simulink model "Adjustable_InputVoltage_Inverter"  (R2015a)
settings: Solver=ode45  StartTime=0.0  StopTime=1  RelTol=1e-3
libraries: powerlib x27, powerlib_meascontrol x7, simulink x2
settings Model: Creator=Koustubh  LastModifiedBy=Koustubh

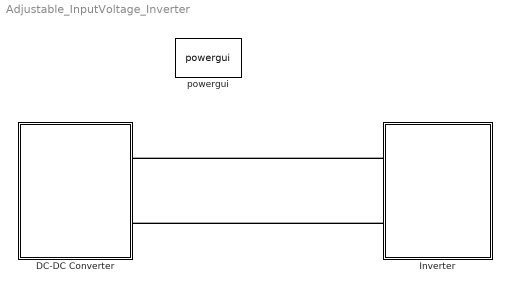
== system Adjustable_InputVoltage_Inverter ==
  DC-DC Converter : Subsystem
  Inverter : Subsystem
  powergui : powerlib/powergui  Priority=1  SimulationMode=Discrete  SolverType=Tustin/Backward Euler (TBE)  SampleTime=50e-6  frequency=60  SPID=off  DisableSnubberDevices=off  DisableRonSwitches=off  DisableVfSwitches=off  SwTol=0  DisplayEquations=off  Interpol=off  methode=off  Ts=100  FunctionMessages=off  echomessages=off  HookPort=off  EnableUseOfTLC=off  x0status=blocks  frequencyindice=0  Pbase=100e6  ErrMax=1e-4  Iterations=50  UnitsV=kV  UnitsW=MW  buscounter=0  RestoreLinks=warning  ResistiveCurrentMeasurement=off  Frange=[0:2:500]  Ylog=off  Xlog=on  ShowGrid=off  save=off  variable=ZData  structure=0  ZoomFFT=off  StartTime=0.0  cycles=1  DisplayStyle=1  fundamental=60  FreqAxis=off  MaxFrequency=1000  frequencyindicesteady=1  RmsSteady=1  display=off
  connections:
  Inverter/LConn1 -- DC-DC Converter/RConn1
  Inverter/LConn2 -- DC-DC Converter/RConn2

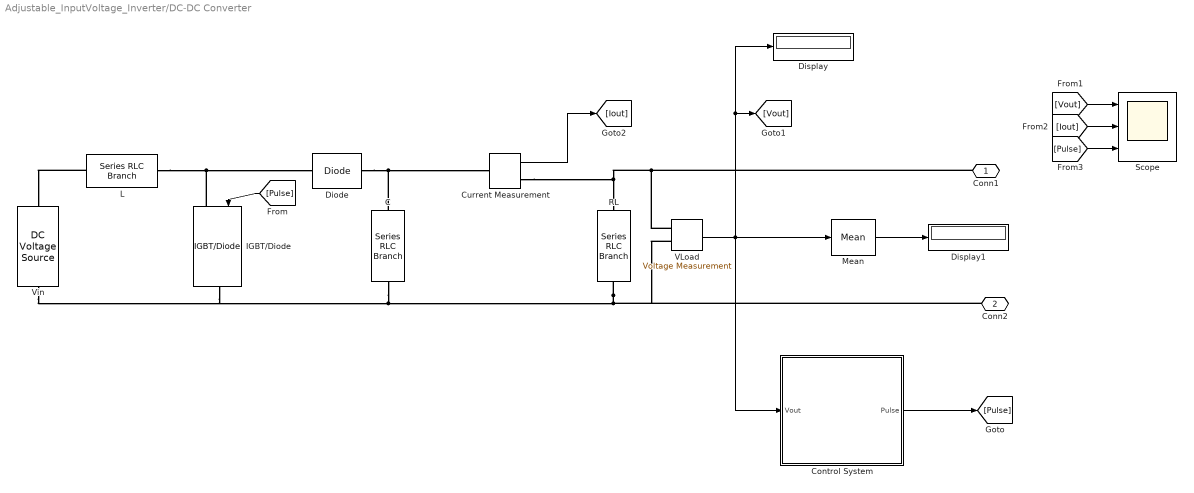
== system Adjustable_InputVoltage_Inverter/DC-DC Converter ==
  C : powerlib/Elements/Series RLC Branch  LConnTagsString=__new0  RConnTagsString=__new0  BranchType=C  Resistance=1  Inductance=1e-3  SetiL0=off  InitialCurrent=0  Capacitance=680e-6  Setx0=off  InitialVoltage=0  Measurements=None
  Control System : Subsystem
  Current Measurement : powerlib/Measurements/Current Measurement  PhasorSimulation=off  OutputType=Complex  PSBequivalent=0
  Diode : powerlib/Power Electronics/Diode  Ron=0.001  Lon=0  Vf=0.8  IC=0  UseSnubber=off  Rs=500  Cs=250e-9  Measurements=off
  Display : Display
  Display1 : Display
  IGBT/Diode : powerlib/Power Electronics/IGBT//Diode  Ron=1e-3  Rs=1e5  Cs=inf  Measurements=off
  L : powerlib/Elements/Series RLC Branch  LConnTagsString=__new0  RConnTagsString=__new0  BranchType=L  Resistance=1  Inductance=60e-6  SetiL0=off  InitialCurrent=0  Capacitance=1e-6  Setx0=off  InitialVoltage=0  Measurements=None
  Mean : powerlib_meascontrol/Measurements/Mean  Freq=60  Vinit=0  Ts=0
  RL : powerlib/Elements/Series RLC Branch  LConnTagsString=__new0  RConnTagsString=__new0  BranchType=R  Resistance=4.8  Inductance=1e-3  SetiL0=off  InitialCurrent=0  Capacitance=1e-6  Setx0=off  InitialVoltage=0  Measurements=None
  Scope : Scope  NumInputPorts=3
      settings: YMin=-5~-5~-5  YMax=5~5~5
  VLoad : powerlib/Measurements/Voltage Measurement  PhasorSimulation=off  OutputType=Complex  PSBequivalent=0
  Vin : powerlib/Electrical Sources/DC Voltage Source  Amplitude=12  Measurements=None
  Conn1 : PMIOPort  Port=1  Side=Right
  Conn2 : PMIOPort  Port=2  Side=Right
  wires:
  VLoad/1 -> Mean/1, Display/1, [Vout], Control System/1(Vout)
  [Pulse] -> IGBT/Diode/1
  Control System/1(Pulse) -> [Pulse]
  [Vout] -> Scope/1
  Current Measurement/1 -> [Iout]
  [Iout] -> Scope/2
  [Pulse] -> Scope/3
  Mean/1 -> Display1/1
  connections:
  RL/RConn1 -- IGBT/Diode/RConn1 -- Vin/LConn1 -- C/RConn1 -- VLoad/LConn2 -- Conn2/RConn1
  C/LConn1 -- Current Measurement/LConn1 -- Diode/RConn1
  Conn1/RConn1 -- Current Measurement/RConn1 -- RL/LConn1 -- VLoad/LConn1
  L/LConn1 -- Vin/RConn1
  L/RConn1 -- IGBT/Diode/LConn1 -- Diode/LConn1

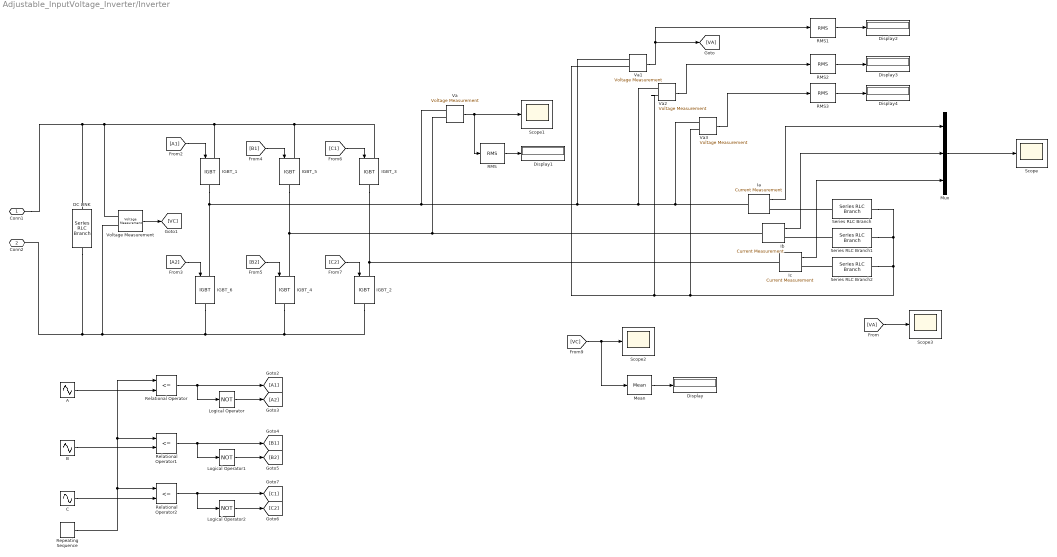
== system Adjustable_InputVoltage_Inverter/Inverter ==
  A : Sin  Frequency=2*pi*50  SampleTime=0
  B : Sin  Frequency=2*pi*50  Phase=120*pi/180  SampleTime=0
  C : Sin  Frequency=2*pi*50  Phase=240*pi/180  SampleTime=0
  "DC LINK " : powerlib/Elements/Series RLC Branch  LConnTagsString=__new0  RConnTagsString=__new0  BranchType=C  Resistance=1  Inductance=1e-3  SetiL0=off  InitialCurrent=0  Capacitance=4700e-6  Setx0=off  InitialVoltage=0  Measurements=None
  Display{,1..4} (5 alike) : Display
  IGBT_{1..6} (6 alike) : powerlib/Power Electronics/IGBT  Ron=0.001  Lon=0  Vf=1  Tf=1e-6  Tt=2e-6  IC=0  Rs=1e5  Cs=inf  Measurements=off
  Ia : powerlib/Measurements/Current Measurement  PhasorSimulation=off  OutputType=Complex  PSBequivalent=0
  Ib : powerlib/Measurements/Current Measurement  PhasorSimulation=off  OutputType=Complex  PSBequivalent=0
  Ic : powerlib/Measurements/Current Measurement  PhasorSimulation=off  OutputType=Complex  PSBequivalent=0
  Logical Operator : Logic  Operator=NOT  AllPortsSameDT=off  OutDataTypeStr=boolean
  Logical Operator1 : Logic  Operator=NOT  AllPortsSameDT=off  OutDataTypeStr=boolean
  Logical Operator2 : Logic  Operator=NOT  AllPortsSameDT=off  OutDataTypeStr=boolean
  Mean : powerlib_meascontrol/Measurements/Mean  Freq=60  Vinit=0  Ts=0
  Mux : Mux  Inputs=3
  RMS{,1..3} (4 alike) : powerlib_meascontrol/Measurements/RMS  TrueRMS=on  Freq=60  RMSInit=120  Ts=0
  Relational Operator : RelationalOperator  Operator=<=  OutDataTypeStr=boolean
  Relational Operator1 : RelationalOperator  Operator=<=  OutDataTypeStr=boolean
  Relational Operator2 : RelationalOperator  Operator=<=  OutDataTypeStr=boolean
  Repeating Sequence : simulink/Sources/Repeating Sequence  rep_seq_t=[0 1/62500]  rep_seq_y=[-1 1]
  Scope{,1..3} (4 alike) : Scope
      Scope settings: YMin=-1  YMax=1.1
      Scope1 settings: YMin=-125  YMax=200  SaveName=ScopeData2
      Scope2 settings: SaveName=ScopeData3
      Scope3 settings: YMin=-1  YMax=1.1  SaveName=ScopeData4
  Series RLC Branch : powerlib/Elements/Series RLC Branch  LConnTagsString=__new0  RConnTagsString=__new0  BranchType=RL  Resistance=5  Inductance=5e-3  SetiL0=off  InitialCurrent=0  Capacitance=1e-6  Setx0=off  InitialVoltage=0  Measurements=None
  Series RLC Branch1 : powerlib/Elements/Series RLC Branch  LConnTagsString=__new0  RConnTagsString=__new0  BranchType=RL  Resistance=5  Inductance=5e-3  SetiL0=off  InitialCurrent=0  Capacitance=1e-6  Setx0=off  InitialVoltage=0  Measurements=None
  Series RLC Branch2 : powerlib/Elements/Series RLC Branch  LConnTagsString=__new0  RConnTagsString=__new0  BranchType=RL  Resistance=5  Inductance=5e-3  SetiL0=off  InitialCurrent=0  Capacitance=1e-6  Setx0=off  InitialVoltage=0  Measurements=None
  Va{,1..3} (4 alike) : powerlib/Measurements/Voltage Measurement  PhasorSimulation=off  OutputType=Complex  PSBequivalent=0
  Voltage Measurement : powerlib/Measurements/Voltage Measurement  PhasorSimulation=off  OutputType=Complex  PSBequivalent=0
  Conn1 : PMIOPort  Port=1  Side=Left
  Conn2 : PMIOPort  Port=2  Side=Left
  wires:
  Relational Operator/1 -> [A1], Logical Operator/1
  Relational Operator1/1 -> [B1], Logical Operator1/1
  Relational Operator2/1 -> [C1], Logical Operator2/1
  Logical Operator/1 -> [A2]
  Logical Operator1/1 -> [B2]
  Logical Operator2/1 -> [C2]
  [A1] -> IGBT_1/1
  [A2] -> IGBT_6/1
  [B2] -> IGBT_4/1
  [C2] -> IGBT_2/1
  [B1] -> IGBT_5/1
  [C1] -> IGBT_3/1
  Repeating Sequence/1 -> Relational Operator2/1, Relational Operator1/1, Relational Operator/1
  A/1 -> Relational Operator/2
  B/1 -> Relational Operator1/2
  C/1 -> Relational Operator2/2
  Ic/1 -> Mux/3
  Ib/1 -> Mux/2
  Ia/1 -> Mux/1
  Mux/1 -> Scope/1
  Voltage Measurement/1 -> [VC]
  [VC] -> Mean/1, Scope2/1
  Mean/1 -> Display/1
  Va/1 -> RMS/1, Scope1/1
  RMS/1 -> Display1/1
  Va1/1 -> [VA], RMS1/1
  RMS1/1 -> Display2/1
  Va2/1 -> RMS2/1
  RMS2/1 -> Display3/1
  RMS3/1 -> Display4/1
  Va3/1 -> RMS3/1
  [VA] -> Scope3/1
  connections:
  IGBT_1/RConn1 -- Va3/LConn1 -- Ia/LConn1 -- Va2/LConn1 -- Va1/LConn1 -- Va/LConn1 -- IGBT_6/LConn1
  IGBT_5/RConn1 -- Va/LConn2 -- Ib/LConn1 -- IGBT_4/LConn1
  IGBT_3/RConn1 -- IGBT_2/LConn1 -- Ic/LConn1
  "DC LINK "/RConn1 -- Voltage Measurement/LConn2 -- IGBT_2/RConn1 -- IGBT_4/RConn1 -- IGBT_6/RConn1 -- Conn2/RConn1
  IGBT_3/LConn1 -- Conn1/RConn1 -- "DC LINK "/LConn1 -- Voltage Measurement/LConn1 -- IGBT_1/LConn1 -- IGBT_5/LConn1
  Series RLC Branch1/RConn1 -- Series RLC Branch/RConn1 -- Va3/LConn2 -- Va2/LConn2 -- Va1/LConn2 -- Series RLC Branch2/RConn1
  Series RLC Branch/LConn1 -- Ia/RConn1
  Series RLC Branch1/LConn1 -- Ib/RConn1
  Series RLC Branch2/LConn1 -- Ic/RConn1

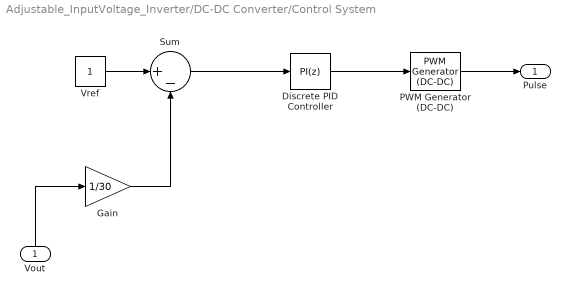
== system Adjustable_InputVoltage_Inverter/DC-DC Converter/Control System ==
  Vout : Inport
  Discrete PID Controller : simulink/Continuous/PID Controller  Controller=PI  TimeDomain=Discrete-time  SampleTime=50e-6  IntegratorMethod=Forward Euler  FilterMethod=Forward Euler  Form=Parallel  UseFilter=on  ControllerParametersSource=internal  P=0.25  I=40  D=0  N=100  InitialConditionSource=internal  InitialConditionForIntegrator=0  InitialConditionForFilter=0  ExternalReset=none  LimitOutput=on  UpperSaturationLimit=0.95  LowerSaturationLimit=0.1  LinearizeAsGain=off  AntiWindupMode=none  Kb=1  TrackingMode=off  Kt=1  PParamMin=[]  PParamMax=[]  IParamMin=[]  IParamMax=[]  DParamMin=[]  DParamMax=[]  NParamMin=[]  NParamMax=[]  KbParamMin=[]  KbParamMax=[]  KtParamMin=[]  KtParamMax=[]  POutMin=[]  POutMax=[]  IOutMin=[]  IOutMax=[]  DOutMin=[]  DOutMax=[]  NOutMin=[]  NOutMax=[]  KbOutMin=[]  KbOutMax=[]  KtOutMin=[]  KtOutMax=[]  IntegratorOutMin=[]  IntegratorOutMax=[]  FilterOutMin=[]  FilterOutMax=[]  SumOutMin=[]  SumOutMax=[]  SumI1OutMin=[]  SumI1OutMax=[]  SumI2OutMin=[]  SumI2OutMax=[]  SumI3OutMin=[]  SumI3OutMax=[]  SumDOutMin=[]  SumDOutMax=[]  SaturationOutMin=[]  SaturationOutMax=[]  IntegratorContinuousStateAttributes=''  IntegratorStateMustResolveToSignalObject=off  IntegratorRTWStateStorageClass=Auto  FilterContinuousStateAttributes=''  FilterStateMustResolveToSignalObject=off  FilterRTWStateStorageClass=Auto  DifferentiatorICPrevScaledInput=0  DifferentiatorOutMin=[]  DifferentiatorOutMax=[]
  Gain : Gain  Gain=1/30
  PWM Generator (DC-DC) : powerlib_meascontrol/Pulse & Signal Generators/PWM Generator (DC-DC)  Fsw=5000  Ts=0
  Sum : Sum  Inputs=|+-
  Vref : Constant
  Pulse : Outport
  wires:
  Vout/1 -> Gain/1
  Vref/1 -> Sum/1
  Sum/1 -> Discrete PID Controller/1
  PWM Generator (DC-DC)/1 -> Pulse/1
  Gain/1 -> Sum/2
  Discrete PID Controller/1 -> PWM Generator (DC-DC)/1
